simulink model "PLUTO_display"  (R2019a)
settings: Solver=FixedStepDiscrete  StartTime=0.0  StopTime=inf  RelTol=1e-3
undefined symbols (not defined in the file or in its folder): Fs, ip, usb
libraries: plutoradiolib x1
settings Model: ModifiedComment=longt -- Fri Jul 26 10:36:19 2019 -- Version 1.25  Creator=longt  LastModifiedBy=longt
settings DataIOCC: SaveOutput=off  SignalLogging=off  DSMLogging=off  SaveTime=off  ReturnWorkspaceOutputs=off

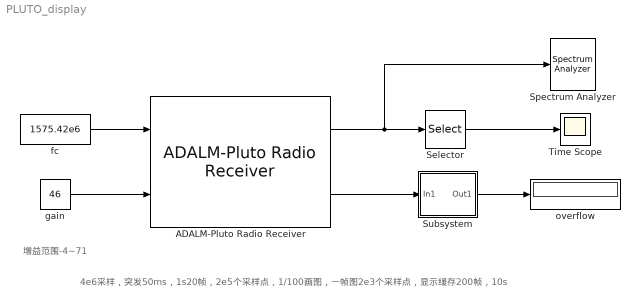
== system PLUTO_display ==
  note: 4e6采样，突发50ms，1s20帧，2e5个采样点，1/100画图，一帧图2e3个采样点，显示缓存200帧，10s
  note: 增益范围-4~71
  ADALM-Pluto Radio Receiver : plutoradiolib/ADALM-Pluto Radio Receiver  RadioID=usb:0  uri=ip:10.0.0.200  CenterFrequencySource=Input Port  CenterFrequency=2.4e9  GainSource=AGC Slow Attack  GainSourceBlock=Input Port  Gain=10  ChannelMapping=1  BasebandSampleRate=4e6  OutputDataType=int16  SamplesPerFrame=2e5  OverflowOutputPort=on  EnableBurstMode=on  NumFramesInBurst=1  ShowAdvancedProperties=off  UseCustomFilter=off  filtPathRates=[737280000 11520000 3840000 1920000 960000 240000]  filtCoefficients=[-192 82 85 -215 228 -102 -110 290 -318 145 160 -426 471 -215 -238 633 -697 318 349 -923 1009 -457 -498 1309 -1423 640 693 -1812 1959 -876 -945 2458 -2647 1180 1268 -3290 3534 -1572 -1688 4375 -4698 2091 2247 -5836 6284 -2807 -3031 7918 -8588 3870 4225 -11182 12324 -5662 -6330 17255 -19735 9507 11312 -33568 43355 -25227 -42139 305542 305542 -42139 -25227 43355 -33568 11312 9507 -19735 17255 -6330 -5662 12324 -11182 4225 3870 -8588 7918 -3031 -2807 6284 -5836 2247 2091 -4698 4375 -1688 -1572 3534 -3290 1268 1180 -2647 2458 -945 -876 1959 -1812 693 640 -1423 1309 -498 -457 1009 -923 349 318 -697 633 -238 -215 471 -426 160 145 -318 290 -110 -102 228 -215 85 82 -192]  filtCoefficientSize=128  filtDecimInterpFactor=4  filtGain=-12  filtRFBandwidth=18000000  filterConfigStruct=struct()  EnableQuadratureCorrection=on  EnableRFDCCorrection=on  EnableBasebandDCCorrection=on  FrequencyCorrection=0  OverrideSampleTime=off  SampleTime=0.02  DataTimeout=Inf  ENSMPinControlMode=None  BISTLoopbackMode=Disabled  BISTToneInject=Disabled  BISTSignalGen=PRBS  BISTToneFreq=Fs/32  BISTToneLevel=0
      settings: SourceProductName=Communications Toolbox Support Package for Analog Devices ADALM-Pluto Radio  SourceProductBaseCode=PLUTO
  Selector : Selector  NumberOfDimensions=2  InputPortWidth=2  IndexOptions=Index vector (dialog),Index vector (dialog)  Indices=(1:2000)*100,1  OutputSizes=1,1
  Spectrum Analyzer : SpectrumAnalyzer
  Subsystem : Subsystem
  Time Scope : Scope
  fc : Constant  Value=1575.42e6  OutMin=325e6  OutMax=3800e6
  gain : Constant  Value=46  OutMin=-4  OutMax=71
  overflow : Display
  wires:
  fc/1 -> ADALM-Pluto Radio Receiver/1
  gain/1 -> ADALM-Pluto Radio Receiver/2
  Subsystem/1(Out1) -> overflow/1
  ADALM-Pluto Radio Receiver/2 -> Subsystem/1(In1)
  ADALM-Pluto Radio Receiver/1 -> Spectrum Analyzer/1, Selector/1
  Selector/1 -> Time Scope/1

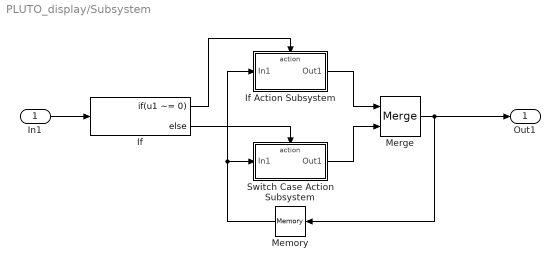
== system PLUTO_display/Subsystem ==
  In1 : Inport
  If : If  IfExpression=u1 ~= 0
  If Action Subsystem : Subsystem  TreatAsAtomicUnit=on
  Memory : Memory
  Merge : Merge
  Switch Case Action Subsystem : Subsystem  TreatAsAtomicUnit=on
  Out1 : Outport
  wires:
  Switch Case Action Subsystem/1(Out1) -> Merge/2
  If Action Subsystem/1(Out1) -> Merge/1
  Merge/1 -> Out1/1, Memory/1
  Memory/1 -> Switch Case Action Subsystem/1(In1), If Action Subsystem/1(In1)
  In1/1 -> If/1
  If/1 -> If Action Subsystem/Action
  If/2 -> Switch Case Action Subsystem/Action

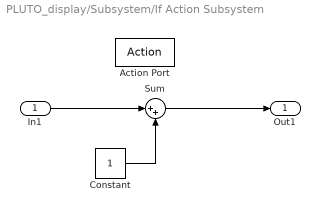
== system PLUTO_display/Subsystem/If Action Subsystem ==
  In1 : Inport
  Action Port : ActionPort  ActionPortLabel=if(u1 ~= 0)
  Constant : Constant
  Sum : Sum  Inputs=|++
  Out1 : Outport
  wires:
  Sum/1 -> Out1/1
  In1/1 -> Sum/1
  Constant/1 -> Sum/2

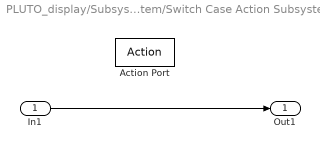
== system PLUTO_display/Subsystem/Switch Case Action Subsystem ==
  In1 : Inport
  Action Port : ActionPort  ActionPortLabel=else
  Out1 : Outport
  wires:
  In1/1 -> Out1/1
